simulink model "Env_cpl_buck"  (R2023b)
settings: Solver=VariableStepAuto  StartTime=0.0  StopTime=0.4  FixedStep=0.001  RelTol=1e-3
PostLoadFcn:
  | , if any(exist('dsrtsu_mdlpostloadfcn', 'file') == [2, 3, 6]), try dsrtsu_mdlpostloadfcn('Execute', bdroot); catch fprintf('Error in PostLoadFcn (dsrtsu_mdlpostloadfcn) for model "%s":\n %s\n', bdroot, lasterr); end, end,
undefined symbols (not defined in the file or in its folder): R
libraries: spsSeriesRLCBranchLib x3, simulink x2, spsControlledCurrentSourceLib x1, spsControlledVoltageSourceLib x1, spsCurrentMeasurementLib x1, spsDiodeLib x1, spsMosfetLib x1, spsVoltageMeasurementLib x1, spsPWMGeneratorDCDCLib x1, rllib x1, spspowerguiLib x1
(part 1 of 4)
Description:
  | Standard RTI1006 template.
  | Supported MATLAB version:  R2019a.
settings Model: Tag=RTI1006  DSRTSU_INTERNAL_RTI_VER=540  DSRTSU_INTERNAL_RTI_TYPE=rti1006  RTICANMMDATA=struct('GeneralSetupData',struct('modelroot','E:\WORK\MigrationScripts','generalsettings',struct('filesettings',struct('destfolder',struct('Name','RTICANMM_FILES','Check',1),'buildfolder',struct('Name','.','Check',1),'AbsDestfolder',struct('Name','E:\WORK\MigrationScripts\RTICANMM_FILES'),'AbsBuildfolder',struct('Name','E:\WORK\MigrationScripts'))),'options',struct('addpaths',1,'rmpaths',1,'addtrcexclusion',logical(1),'cannavigator',struct('checkmonitoring',0),'show_usrtrc',0,'use_usrtrc',0),'advanced',struct('options',ones(1,100)),'MPSetup',{{}},'RTI',struct('Type','RTI1006','Ver','7.12','Date','02-May-2019'),'modelname','','block','untitled'))  DSRTSU_INTERNAL_RTIFPGA=130  Creator=user  LastModifiedBy=Dean
settings SolverCC: AlgebraicLoopSolver=TrustRegion
settings DataIOCC: ReturnWorkspaceOutputs=off
settings OptimizationCC: BlockReduction=off  OptimizeBlockIOStorage=off  BufferReuse=off  GlobalBufferReuse=off  ExpressionFolding=off  LocalBlockOutputs=off  OptimizeDataStoreBuffers=off  BusAssignmentInplaceUpdate=off
settings DebuggingCC: UnconnectedInputMsg=warning  UnconnectedOutputMsg=warning  UnconnectedLineMsg=warning  PregeneratedLibrarySubsystemCodeDiagnostic=none  ArithmeticOperatorsInVariantConditions=warning
settings HardwareCC: ProdBitPerPointer=32  ProdBitPerSizeT=32  ProdBitPerPtrDiffT=32  ProdLargestAtomicInteger=Integer  ProdWordSize=32  ProdHWDeviceType=Custom Processor->Custom  TargetIntDivRoundTo=Zero  TargetEndianess=LittleEndian  TargetHWDeviceType=Custom Processor->Custom
settings ModelReferenceCC: EnableRefExpFcnMdlSchedulingChecks=on
settings SFSimCC: SimUseLocalCustomCode=off  MATLABDynamicMemAlloc=off  CustomCodeUndefinedFunction=UseInterfaceOnly
settings RTWCC: Description=dSPACE DS1006 Hardware Platform  SystemTargetFile=rti1006.tlc  MakeCommand=make_rti  TemplateMakefile=rti1006.tmf  RTWUseLocalCustomCode=off  DLArmComputeVersion=19.05
settings CodeAppCC: StateflowObjectComments=on
settings STFCustomTargetCC: TargetLangStandard=C89/C90 (ANSI)  ParMdlRefBuildCompliant=on  MatFileLogging=on  SystemTargetFile=rti1006.tlc
settings GRTTargetCC: TargetLangStandard=C89/C90 (ANSI)  CompOptLevelCompliant=off  ConcurrentExecutionCompliant=off  CombineOutputUpdateFcns=off  CPPClassGenCompliant=off  UseToolchainInfoCompliant=off
settings ConfigComp: CovMetricSettings=dswe

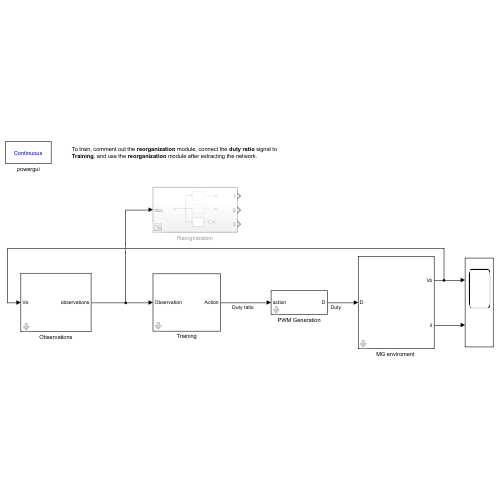
[thumbnail: Simulink's stored preview of the top-level diagram]
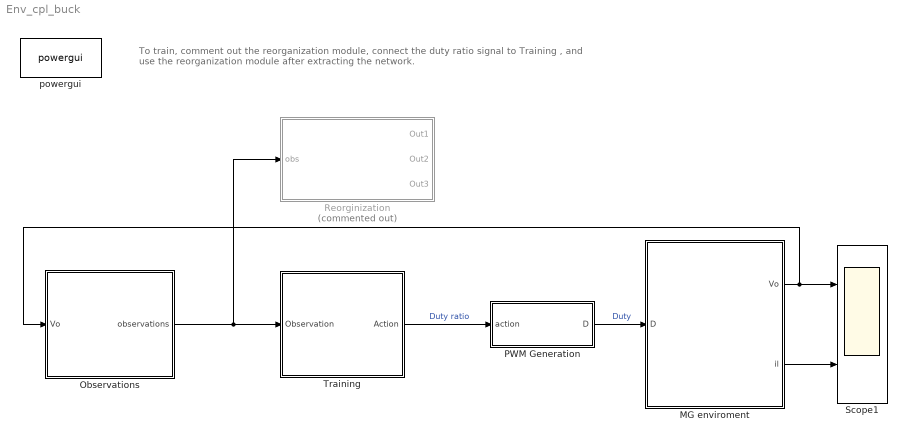
== system Env_cpl_buck ==
  note: To train, comment out the reorganization module, connect the duty ratio signal to Training , and use the reorganization module after extracting the network.
  "MG enviroment " : Subsystem  mask{E=200, L=1e-3, C=1e-3, t1=0.14, t2=0.2, p1=200, p2=800}
      mask prompts: E "Input voltage E (V)"; L "L (H)"; C "C (F)"; t1 "Step time 1"; t2 "Step time2"; p1 "Initial power (W)"; p2 "Switched power (W)"
      mask DialogControl ParameterGroupVar Prompt: 参数
  Observations : Subsystem  mask{Vref=100}
      mask DialogControl DescTextVar Prompt: Voltage reference
      mask DialogControl ParameterGroupVar Prompt: 参数
  PWM Generation : Subsystem  mask{fsw=2e4}
      mask prompts: fsw "Switching frequency (Hz)"
      mask DialogControl ParameterGroupVar Prompt: 参数
  Reorginization : Subsystem  Commented=on
  Scope1 : Scope  NumInputPorts=2
  Training : Subsystem  mask{beta1=9, beta2=1, beta3=10}
      mask DialogControl DescTextVar Prompt: Reward and penalty parameters
      mask DialogControl ParameterGroupVar Prompt: 参数
  powergui : spspowerguiLib/powergui  Priority=1  SimulationMode=Continuous  SampleTime=50e-6  frequency=60  Iterations=50  frequencyindice=0  Pbase=100e6  ErrMax=1e-4  UnitsV=kV  UnitsW=MW  buscounter=0  FunctionMessages=off  echomessages=off  EnableUseOfTLC=off  CurrentSourceSwitches=off  DisableSnubberDevices=off  DisableRonSwitches=off  DisableVfSwitches=off  DisplayEquations=off  AutomaticDiscreteSolvers=off  SolverType=Tustin/Backward Euler (TBE)  Interpol=off  ExternalGateDelay=off  methode=off  Ts=100  x0status=blocks  SPID=on  SwTol=0  HookPort=off  NonlinearTolerance=0  nMaxIteration=15  ContinueOnMaxIteration=off  RestoreLinks=warning  ResistiveCurrentMeasurement=off  Frange=[0:2:500]  Ylog=off  Xlog=on  ShowGrid=off  save=off  variable=ZData  structure=0  ZoomFFT=off  StartTime=0.0  cycles=1  DisplayStyle=1  fundamental=60  FreqAxis=off  MaxFrequency=1000  frequencyindicesteady=1  RmsSteady=1  display=off
  wires:
  Observations/1(observations) -> Reorginization/1(obs), Training/1(Observation)
  "MG enviroment "/1(Vo) -> Observations/1(Vo), Scope1/1
  PWM Generation/1(D) -> "MG enviroment "/1(D)  "Duty"
  "MG enviroment "/2(il) -> Scope1/2
  Training/1(Action) -> PWM Generation/1(action)  "Duty ratio"

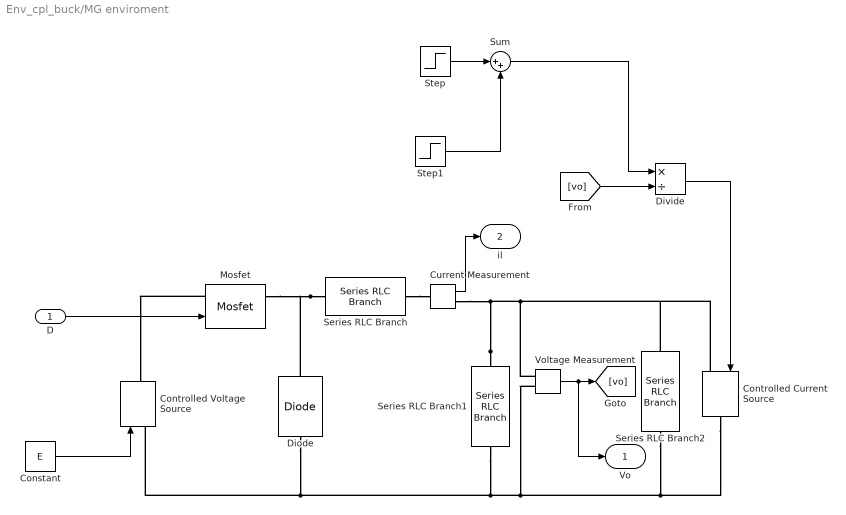
== system Env_cpl_buck/MG enviroment  ==
  D : Inport
  Constant : Constant  Value=E
  Controlled Current Source : spsControlledCurrentSourceLib/Controlled Current Source  Initialize=on  Source_Type=AC  Amplitude=0  Phase=0  Frequency=0  Measurements=None
  Controlled Voltage Source : spsControlledVoltageSourceLib/Controlled Voltage Source  Initialize=on  Source_Type=AC  Amplitude=0  Phase=0  Frequency=0  Measurements=None
  Current Measurement : spsCurrentMeasurementLib/Current Measurement  PhasorSimulation=off  OutputType=Complex  PSBequivalent=0
  Diode : spsDiodeLib/Diode  Ron=0.001  Lon=0  Vf=0.8  IC=0  UseSnubber=0  Rs=500  Cs=250e-9  Measurements=off
  Divide : Product  Inputs=*/
  Mosfet : spsMosfetLib/Mosfet  Ron=0.1  Lon=0  Rd=0.01  Vfd=0  IC=0  Rs=1e5  Cs=inf  Measurements=on
  Series RLC Branch : spsSeriesRLCBranchLib/Series RLC Branch  LConnTagsString=__new0  RConnTagsString=__new0  BranchType=L  Resistance=1  Inductance=L  SetiL0=off  InitialCurrent=0  Capacitance=1e-6  Setx0=off  InitialVoltage=0  Measurements=None
  Series RLC Branch1 : spsSeriesRLCBranchLib/Series RLC Branch  LConnTagsString=__new0  RConnTagsString=__new0  BranchType=C  Resistance=1  Inductance=0.002  SetiL0=off  InitialCurrent=0  Capacitance=C  Setx0=on  InitialVoltage=100  Measurements=None
  Series RLC Branch2 : spsSeriesRLCBranchLib/Series RLC Branch  LConnTagsString=__new0  RConnTagsString=__new0  BranchType=R  Resistance=150000  Inductance=R  SetiL0=off  InitialCurrent=0  Capacitance=1e-6  Setx0=off  InitialVoltage=0  Measurements=None
  Step : Step  Time=t1  Before=p1  After=p2  SampleTime=0
  Step1 : Step  Time=t2  After=p1-p2  SampleTime=0
  Sum : Sum  Inputs=|++
  Voltage Measurement : spsVoltageMeasurementLib/Voltage Measurement  PhasorSimulation=off  OutputType=Complex  PSBequivalent=0
  Vo : Outport  VectorParamsAs1DForOutWhenUnconnected=off
  il : Outport  Port=2  VectorParamsAs1DForOutWhenUnconnected=off
  wires:
  D/1 -> Mosfet/1
  Current Measurement/1 -> il/1
  Voltage Measurement/1 -> Vo/1, [vo]
  Divide/1 -> Controlled Current Source/1
  Constant/1 -> Controlled Voltage Source/1
  [vo] -> Divide/2
  Step1/1 -> Sum/2
  Step/1 -> Sum/1
  Sum/1 -> Divide/1
  connections:
  Controlled Current Source/RConn1 -- Diode/LConn1 -- Controlled Voltage Source/LConn1 -- Series RLC Branch1/RConn1 -- Voltage Measurement/LConn2 -- Series RLC Branch2/RConn1
  Series RLC Branch1/LConn1 -- Current Measurement/RConn1 -- Series RLC Branch2/LConn1 -- Controlled Current Source/LConn1 -- Voltage Measurement/LConn1
  Series RLC Branch/LConn1 -- Mosfet/RConn1 -- Diode/RConn1
  Series RLC Branch/RConn1 -- Current Measurement/LConn1
  Mosfet/LConn1 -- Controlled Voltage Source/RConn1

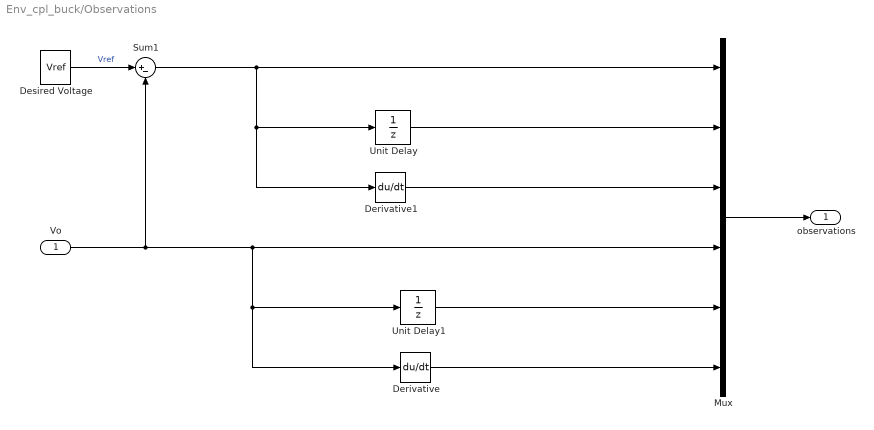
== system Env_cpl_buck/Observations ==
  Vo : Inport
  Derivative : Derivative
  Derivative1 : Derivative
  Desired Voltage : Constant  Value=Vref
  Mux : Mux  Inputs=6
  Sum1 : Sum  Inputs=|+-  SaturateOnIntegerOverflow=on
  Unit Delay : UnitDelay  SampleTime=-1  HasFrameUpgradeWarning=on
  Unit Delay1 : UnitDelay  SampleTime=-1  HasFrameUpgradeWarning=on
  observations : Outport  VectorParamsAs1DForOutWhenUnconnected=off
  wires:
  Mux/1 -> observations/1
  Derivative1/1 -> Mux/3
  Unit Delay/1 -> Mux/2
  Derivative/1 -> Mux/6
  Unit Delay1/1 -> Mux/5
  Vo/1 -> Sum1/2, Unit Delay1/1, Derivative/1, Mux/4
  Sum1/1 -> Unit Delay/1, Derivative1/1, Mux/1
  Desired Voltage/1 -> Sum1/1  "Vref"

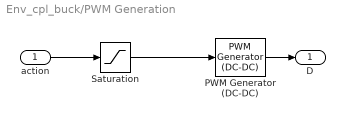
== system Env_cpl_buck/PWM Generation ==
  action : Inport
  PWM Generator (DC-DC) : spsPWMGeneratorDCDCLib/PWM Generator (DC-DC)  Fsw=fsw  Ts=0
  Saturation : Saturate  UpperLimit=0.99  LowerLimit=0.01
  D : Outport  VectorParamsAs1DForOutWhenUnconnected=off
  wires:
  PWM Generator (DC-DC)/1 -> D/1
  Saturation/1 -> PWM Generator (DC-DC)/1
  action/1 -> Saturation/1

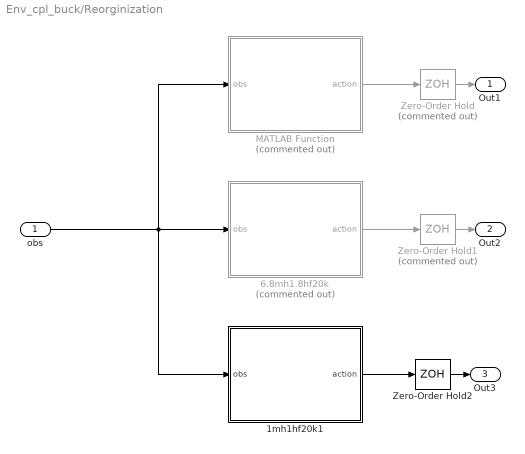
== system Env_cpl_buck/Reorginization ==
  obs : Inport
  1mh1hf20k1 : MATLAB Function  TreatAsAtomicUnit=on
  6.8mh1.8hf20k : MATLAB Function  Commented=on  TreatAsAtomicUnit=on
  MATLAB Function : MATLAB Function  Commented=on  TreatAsAtomicUnit=on
  Zero-Order Hold : ZeroOrderHold  Commented=on  SampleTime=1/20000
  Zero-Order Hold1 : ZeroOrderHold  Commented=on  SampleTime=1/20000
  Zero-Order Hold2 : ZeroOrderHold  SampleTime=1/20000
  Out1 : Outport
  Out2 : Outport  Port=2
  Out3 : Outport  Port=3
  wires:
  obs/1 -> MATLAB Function/1(obs), 1mh1hf20k1/1(obs), 6.8mh1.8hf20k/1(obs)
  Zero-Order Hold1/1 -> Out2/1
  MATLAB Function/1(action) -> Zero-Order Hold/1
  6.8mh1.8hf20k/1(action) -> Zero-Order Hold1/1
  1mh1hf20k1/1(action) -> Zero-Order Hold2/1
  Zero-Order Hold/1 -> Out1/1
  Zero-Order Hold2/1 -> Out3/1

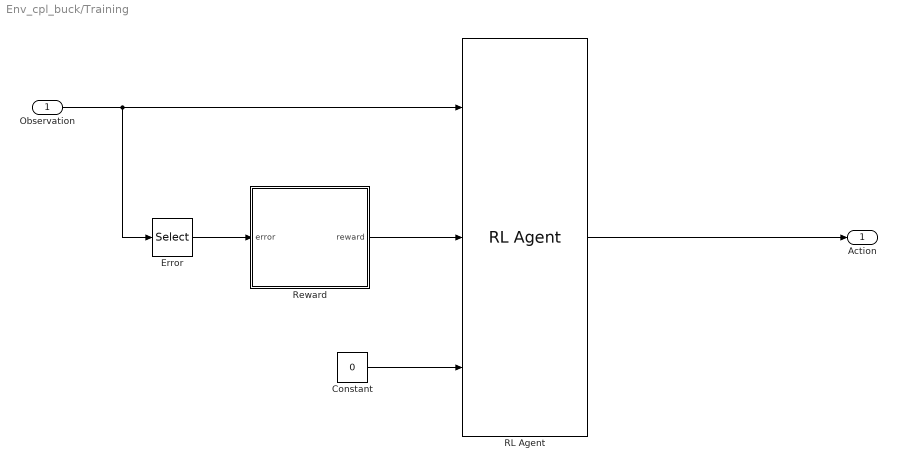
== system Env_cpl_buck/Training ==
  Observation : Inport
  Constant : Constant  Value=0
  Error : Selector  InputPortWidth=6  IndexOptions=Index vector (dialog)  Indices=[1]  OutputSizes=1
  RL Agent : rllib/RL Agent  Agent=agent  ExternalActionAsInput=off  ProvideLastAction=off  ProvideCumRwd=off  TreatAsDirectFeedthrough=on  UseStrictObservationDataTypes=off
  Reward : Subsystem
  Action : Outport
  wires:
  Constant/1 -> RL Agent/3
  RL Agent/1 -> Action/1
  Reward/1(reward) -> RL Agent/2
  Error/1 -> Reward/1(error)
  Observation/1 -> Error/1, RL Agent/1

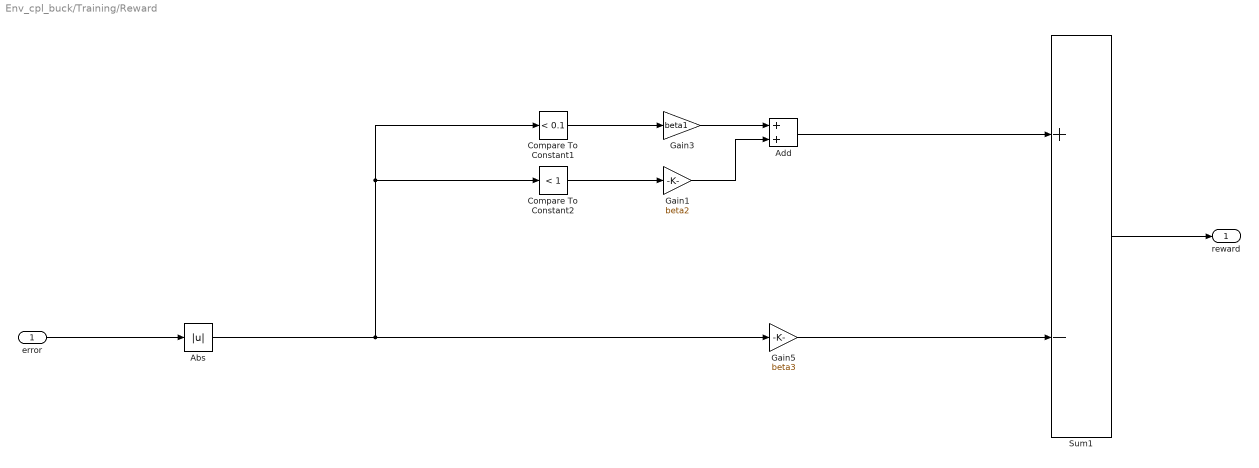
== system Env_cpl_buck/Training/Reward ==
  error : Inport
  Abs : Abs  SaturateOnIntegerOverflow=off
  Add : Sum
  Compare To Constant1 : simulink/Logic and Bit Operations/Compare To Constant  relop=<  const=0.1  OutDataTypeStr=boolean
  Compare To Constant2 : simulink/Logic and Bit Operations/Compare To Constant  relop=<  const=1  OutDataTypeStr=boolean
  Gain1 : Gain  Gain=beta2
  Gain3 : Gain  Gain=beta1
  Gain5 : Gain  Gain=beta3
  Sum1 : Sum  Inputs=+-  OutDataTypeStr=double
  reward : Outport  VectorParamsAs1DForOutWhenUnconnected=off
  wires:
  Compare To Constant1/1 -> Gain3/1
  Gain3/1 -> Add/1
  Abs/1 -> Gain5/1, Compare To Constant2/1, Compare To Constant1/1
  Add/1 -> Sum1/1
  Sum1/1 -> reward/1
  error/1 -> Abs/1
  Gain1/1 -> Add/2
  Compare To Constant2/1 -> Gain1/1
  Gain5/1 -> Sum1/2
